simulink model "VoltageControlledResistor"  (R2016a)
settings: Solver=ode3  StartTime=0.0  StopTime=10.0  FixedStep=Ts  RelTol=1e-3
InitFcn:
  | Ts=0.01;
libraries: powerlib x7
settings Model: Creator=ihalatci  LastModifiedBy=Rafi
settings DataIOCC: LimitDataPoints=on  SaveFormat=Array  SignalLoggingSaveFormat=ModelDataLogs
settings OptimizationCC: ExpressionDepthLimit=2147483647  InitFltsAndDblsToZero=on
settings DebuggingCC: SaveWithParameterizedLinksMsg=none  UnderspecifiedInitializationDetection=Classic  MergeDetectMultiDrivingBlocksExec=none  SignalResolutionControl=TryResolveAllWithWarning  SolverPrmCheckMsg=warning  MultiTaskDSMMsg=warning  MultiTaskCondExecSysMsg=none  FcnCallInpInsideContextMsg=UseLocalSettings  StateNameClashWarn=warning
settings HardwareCC: ProdBitPerPointer=32  ProdLargestAtomicFloat=None  ProdIntDivRoundTo=Undefined  ProdEndianess=Unspecified  ProdWordSize=32  ProdHWDeviceType=32-bit Generic
settings ModelReferenceCC: PropagateSignalLabelsOutOfModel=off
settings GRTTargetCC: TargetFcnLib=ansi_tfl_tmw.mat  CombineOutputUpdateFcns=off  GRTInterface=on
settings ConfigComp: CovModelRefEnable=Off

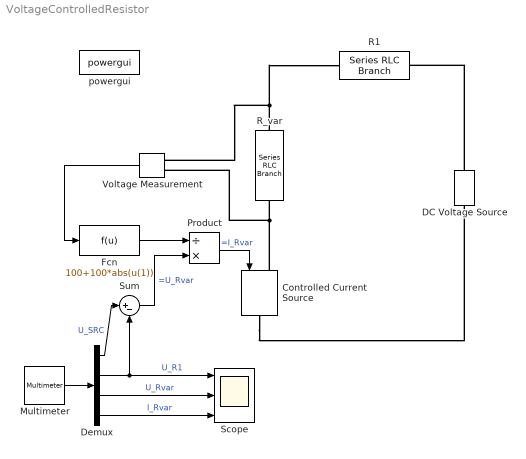
== system VoltageControlledResistor ==
  Controlled Current Source : powerlib/Electrical Sources/Controlled Current Source  Initialize=on  Source_Type=DC  Amplitude=1  Phase=0  Frequency=0  Measurements=Current
  DC Voltage Source : powerlib/Electrical Sources/DC Voltage Source  Amplitude=100  Measurements=Voltage
  Demux : Demux
  Fcn : Fcn  Expr=100+100*abs(u(1))
  Multimeter : powerlib/Measurements/Multimeter  PhasorSimulation=off  OutputType=Complex  sel=[3 1 2 4]  L=5  Gain=[1 1 1 1]  yselected={'Usrc: DC Voltage Source','Ub: R1','Ub: R_var','Ib: R_var'};  PSBOutputType=1  PSBequivalent=0  AxesSetting=[0,0.1,-100,100]  Display=0  SavedBlockNames=-11
  Product : Product  Inputs=/*  RndMeth=Zero
  R1 : powerlib/Elements/Series RLC Branch  LConnTagsString=__new0  RConnTagsString=__new0  BranchType=R  Resistance=100  Inductance=1.0  SetiL0=off  InitialCurrent=0  Capacitance=1.0  Setx0=off  InitialVoltage=0  Measurements=Branch voltage
  R_var : powerlib/Elements/Series RLC Branch  LConnTagsString=__new0  RConnTagsString=__new0  BranchType=R  Resistance=100  Inductance=1.0  SetiL0=off  InitialCurrent=0  Capacitance=1.0  Setx0=off  InitialVoltage=0  Measurements=Branch voltage and current
  Scope : Scope  NumInputPorts=3
  Sum : Sum  Inputs=|+-
  Voltage Measurement : powerlib/Measurements/Voltage Measurement  PhasorSimulation=off  OutputType=Complex  PSBequivalent=0
  powergui : powerlib/powergui  SimulationMode=Continuous  SolverType=Tustin  SampleTime=Ts  frequency=60  SPID=off  DisableSnubberDevices=off  DisableRonSwitches=off  DisableVfSwitches=off  SwTol=0  DisplayEquations=off  Interpol=off  ExternalGateDelay=off  methode=off  Ts=0  FunctionMessages=off  echomessages=off  HookPort=off  EnableUseOfTLC=off  x0status=blocks  frequencyindice=0  Pbase=100e6  ErrMax=1e-4  Iterations=50  UnitsV=kV  UnitsW=MW  buscounter=0  RestoreLinks=warning  ResistiveCurrentMeasurement=off  Frange=[0:2:500]  Ylog=off  Xlog=on  ShowGrid=off  save=off  variable=ZData  structure=0  ZoomFFT=on  StartTime=0.0  cycles=1  DisplayStyle=1  fundamental=60  FreqAxis=off  MaxFrequency=1000  frequencyindicesteady=1  RmsSteady=1  display=off
  wires:
  Product/1 -> Controlled Current Source/1  "=I_Rvar"
  Multimeter/1 -> Demux/1
  Sum/1 -> Product/2  "=U_Rvar"
  Demux/1 -> Sum/1  "U_SRC"
  Demux/2 -> Sum/2, Scope/1  "U_R1"
  Demux/3 -> Scope/2  "U_Rvar"
  Demux/4 -> Scope/3  "I_Rvar"
  Voltage Measurement/1 -> Fcn/1
  Fcn/1 -> Product/1
  connections:
  Controlled Current Source/RConn1 -- DC Voltage Source/LConn1
  DC Voltage Source/RConn1 -- R1/LConn1
  Controlled Current Source/LConn1 -- R_var/RConn1 -- Voltage Measurement/LConn2
  R_var/LConn1 -- R1/RConn1 -- Voltage Measurement/LConn1
